simulink model "powersystemsFinalTest"  (R2023a)
settings: Solver=VariableStepAuto  StartTime=0.0  StopTime=50  RelTol=1e-3
model workspace (MAT data in the model file):
  step = 1
values from neighbouring files (symbols this model uses):
  C_TCSC = 1 / (2*pi*60*Xc)    [Final_TCSC.m]
  final_step = [1,1,1,1]    [Final_TCSC.m]
  L_line = X_line / (2*pi*60)    [Final_TCSC.m]
  L_TCSC = Xl_stage / (2*pi*60)    [Final_TCSC.m]
  R_load = 1000    [Final_TCSC.m]
  Vs = str2double(inputs{1}) * 1e3    [Final_TCSC.m]
libraries: spsSeriesRLCBranchLib x10, spsThyristorLib x8, spsRMSLib x7, spsFourierLib x3, spsVoltageMeasurementLib x3, spsPowerLib x2, spsACVoltageSourceLib x1, aerolibconvert2 x1, spsCurrentMeasurementLib x1, sps_lib x1, spspowerguiLib x1
settings Model: Creator=moham  LastModifiedBy=nonyf
settings DebuggingCC: UnconnectedInputMsg=warning  UnconnectedOutputMsg=warning  UnconnectedLineMsg=warning
settings ModelReferenceCC: EnableRefExpFcnMdlSchedulingChecks=on
settings RTWCC: DLArmComputeVersion=19.05

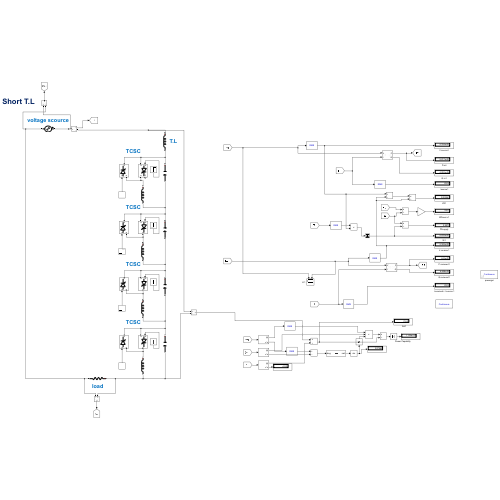
[thumbnail: Simulink's stored preview of the top-level diagram]
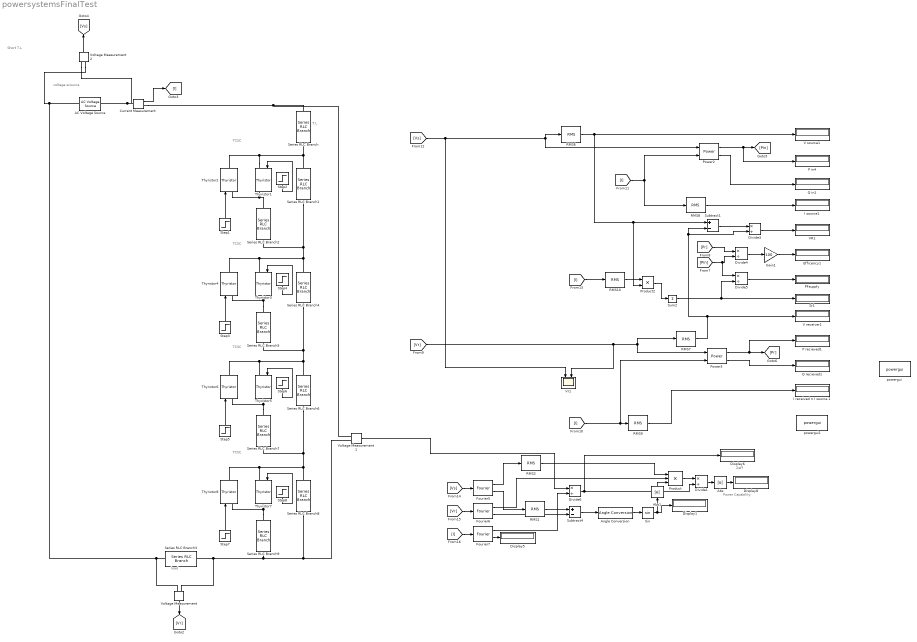
== system powersystemsFinalTest ==
  note: Zeff
  note: load
  note: TCSC
  note: T.L
  note: voltage scource
  note: Short T.L
  note: TCSC
  note: TCSC
  note: TCSC
  note: Power Capability
  AC Voltage Source : spsACVoltageSourceLib/AC Voltage Source  Amplitude=Vs  Phase=0  Frequency=60  SampleTime=0  Measurements=None  BusType=swing  Pref=10e3  Qref=0  Qmin=-inf  Qmax=+inf
  Abs : Abs  SaturateOnIntegerOverflow=off
  Abs1 : Abs  SaturateOnIntegerOverflow=off
  Angle Conversion : aerolibconvert2/Angle Conversion  IU=deg  OU=rad
  Current Measurement : spsCurrentMeasurementLib/Current Measurement  PhasorSimulation=off  OutputType=Complex  PSBequivalent=0
  Display{1,5..6,8} (4 alike) : Display
  Divide{1,3..6} (5 alike) : Product  Inputs=*/
  Efficency1 : Display
  Fourier5 : spsFourierLib/Fourier  Freq=60  n=1  InInit=[0, 0]  Ts=0
  Fourier6 : spsFourierLib/Fourier  Freq=60  n=1  InInit=[0, 0]  Ts=0
  Fourier7 : spsFourierLib/Fourier  Freq=60  n=1  InInit=[0, 0]  Ts=0
  Gain1 : Gain  Gain=100
  I received = I source 1 : Display
  I source1 : Display
  P in4 : Display
  P recieved1 : Display
  PFsupply : Display
  Power2 : spsPowerLib/Power  Freq=60  Vinit=[1, 0]  Iinit=[1, 0]  Ts=0
  Power3 : spsPowerLib/Power  Freq=60  Vinit=[1, 0]  Iinit=[1, 0]  Ts=0
  Product : Product  Inputs=3
  Product2 : Product
  Q in1 : Display
  Q recieved1 : Display
  RMS{1..2,6..10} (7 alike) : spsRMSLib/RMS  TrueRMS=on  Freq=60  RMSInit=120  Ts=0
  Series RLC Branch : spsSeriesRLCBranchLib/Series RLC Branch  LConnTagsString=__new0  RConnTagsString=__new0  BranchType=L  Resistance=50  Inductance=L_line  SetiL0=off  InitialCurrent=0  Capacitance=0  Setx0=off  InitialVoltage=0  Measurements=None
  Series RLC Branch{1,4,6,8} (4 alike) : spsSeriesRLCBranchLib/Series RLC Branch  LConnTagsString=__new0  RConnTagsString=__new0  BranchType=C  Resistance=50  Inductance=0.1327  SetiL0=off  InitialCurrent=0  Capacitance=C_TCSC  Setx0=off  InitialVoltage=0  Measurements=None
  Series RLC Branch{2,5,7,9} (4 alike) : spsSeriesRLCBranchLib/Series RLC Branch  LConnTagsString=__new0  RConnTagsString=__new0  BranchType=L  Resistance=50  Inductance=L_TCSC  SetiL0=off  InitialCurrent=0  Capacitance=0  Setx0=off  InitialVoltage=0  Measurements=None
  Series RLC Branch3 : spsSeriesRLCBranchLib/Series RLC Branch  LConnTagsString=__new0  RConnTagsString=__new0  BranchType=R  Resistance=R_load  Inductance=1.3  SetiL0=off  InitialCurrent=0  Capacitance=0  Setx0=off  InitialVoltage=0  Measurements=None
  Sin : Trigonometry
  Sr1 : Display
  Step1 : Step  Time=5  After=final_step(1)  SampleTime=0
  Step2 : Step  Time=5  After=final_step(1)  SampleTime=0
  Step3 : Step  Time=5  After=final_step(2)  SampleTime=0
  Step4 : Step  Time=5  After=final_step(2)  SampleTime=0  ZeroCross=off
  Step5 : Step  Time=5  After=final_step(3)  SampleTime=0
  Step6 : Step  Time=5  After=final_step(3)  SampleTime=0
  Step7 : Step  Time=5  After=final_step(4)  SampleTime=0
  Step8 : Step  Time=5  After=final_step(4)  SampleTime=0
  Subtract1 : Sum  Inputs=+-
  Subtract4 : Sum  Inputs=+-
  Sum2 : Sum  Inputs=+
  Thyristor1 : spsThyristorLib/Thyristor  Ron=0  Lon=0  Vf=0  IC=0  Rs=0  Cs=0  Measurements=on
  Thyristor{2..8} (7 alike) : spsThyristorLib/Thyristor  Ron=0  Lon=0  Vf=0  IC=0  Rs=0  Cs=0  Measurements=off
  V receiver1 : Display
  V source1 : Display
  VR1 : Display
  Voltage Measurement : spsVoltageMeasurementLib/Voltage Measurement  PhasorSimulation=off  OutputType=Complex  PSBequivalent=0
  Voltage Measurement1 : spsVoltageMeasurementLib/Voltage Measurement  PhasorSimulation=off  OutputType=Complex  PSBequivalent=0
  Voltage Measurement2 : spsVoltageMeasurementLib/Voltage Measurement  PhasorSimulation=off  OutputType=Complex  PSBequivalent=0
  Vr1 : Scope  NumInputPorts=2
  powergui : sps_lib/powergui  Priority=1  SimulationMode=Continuous  SampleTime=50e-6  frequency=60  Iterations=50  frequencyindice=60  Pbase=100e6  ErrMax=1e-4  UnitsV=kV  UnitsW=MW  buscounter=0  FunctionMessages=off  echomessages=off  EnableUseOfTLC=off  CurrentSourceSwitches=off  DisableSnubberDevices=off  DisableRonSwitches=off  DisableVfSwitches=off  DisplayEquations=off  AutomaticDiscreteSolvers=off  SolverType=Tustin/Backward Euler (TBE)  Interpol=off  ExternalGateDelay=off  methode=off  Ts=100  x0status=blocks  SPID=on  SwTol=0  HookPort=off  NonlinearTolerance=1e-4  nMaxIteration=100  ContinueOnMaxIteration=off  RestoreLinks=warning  ResistiveCurrentMeasurement=off  Frange=[0:2:500]  Ylog=off  Xlog=on  ShowGrid=off  save=off  variable=ZData  structure=0  ZoomFFT=off  StartTime=0.0  cycles=1  DisplayStyle=1  fundamental=60  FreqAxis=off  MaxFrequency=1000  frequencyindicesteady=1  RmsSteady=1  display=off
  powergui1 : spspowerguiLib/powergui  Priority=1  SimulationMode=Continuous  SampleTime=50e-6  frequency=60  Iterations=50  frequencyindice=60  Pbase=100e6  ErrMax=1e-4  UnitsV=kV  UnitsW=MW  buscounter=0  FunctionMessages=off  echomessages=off  EnableUseOfTLC=off  CurrentSourceSwitches=off  DisableSnubberDevices=off  DisableRonSwitches=off  DisableVfSwitches=off  DisplayEquations=off  AutomaticDiscreteSolvers=off  SolverType=Tustin/Backward Euler (TBE)  Interpol=off  ExternalGateDelay=off  methode=off  Ts=100  x0status=blocks  SPID=on  SwTol=0  HookPort=off  NonlinearTolerance=1e-4  nMaxIteration=100  ContinueOnMaxIteration=off  RestoreLinks=warning  ResistiveCurrentMeasurement=off  Frange=[0:2:500]  Ylog=off  Xlog=on  ShowGrid=off  save=off  variable=ZData  structure=0  ZoomFFT=off  StartTime=0.0  cycles=1  DisplayStyle=1  fundamental=60  FreqAxis=off  MaxFrequency=1000  frequencyindicesteady=1  RmsSteady=1  display=off
  wires:
  Step1/1 -> Thyristor2/1
  Step2/1 -> Thyristor1/1
  Voltage Measurement/1 -> [Vr]
  Current Measurement/1 -> [I]
  Voltage Measurement2/1 -> [Vs]
  Step3/1 -> Thyristor4/1
  Step4/1 -> Thyristor3/1
  Step6/1 -> Thyristor5/1
  Step5/1 -> Thyristor6/1
  Step8/1 -> Thyristor7/1
  Step7/1 -> Thyristor8/1
  [Vr] -> Fourier6/1
  Fourier7/1 -> Divide6/2
  [I] -> Fourier7/1
  Divide6/1 -> Divide1/2, Display6/1
  [Vs] -> Fourier5/1
  Fourier7/2 -> Display5/1
  Gain1/1 -> Efficency1/1
  Product2/1 -> Sum2/1
  [I] -> Power3/2, RMS9/1
  RMS8/1 -> I source1/1
  Divide3/1 -> VR1/1
  Divide5/1 -> PFsupply/1
  Power3/1 -> P recieved1/1, [Pr]
  RMS10/1 -> Product2/1
  RMS7/1 -> Divide3/2, Subtract1/2, V receiver1/1
  [Pin] -> Divide5/1, Divide4/2
  [Vr] -> RMS7/1, Power3/1, Vr1/2
  RMS9/1 -> I received = I source 1/1
  [Pr] -> Divide4/1
  Power2/1 -> P in4/1, [Pin]
  [I] -> RMS10/1
  Power3/2 -> Q recieved1/1
  Sum2/1 -> Divide5/2, Sr1/1
  Power2/2 -> Q in1/1
  RMS6/1 -> Product2/2, Subtract1/1, V source1/1
  [Vs] -> Power2/1, RMS6/1, Vr1/1
  Subtract1/1 -> Divide3/1
  Divide4/1 -> Gain1/1
  [I] -> RMS8/1, Power2/2
  Fourier5/2 -> RMS1/1
  Fourier6/2 -> Subtract4/2
  Fourier6/1 -> Product/2
  Fourier5/1 -> RMS2/1
  Product/1 -> Divide1/1
  Divide1/1 -> Abs/1
  Abs/1 -> Display8/1
  Voltage Measurement1/1 -> Divide6/1
  Angle Conversion/1 -> Sin/1
  Subtract4/1 -> Angle Conversion/1
  Sin/1 -> Abs1/1, Display1/1
  RMS2/1 -> Product/1
  RMS1/1 -> Subtract4/1
  Abs1/1 -> Product/3
  connections:
  Series RLC Branch4/LConn1 -- Series RLC Branch1/RConn1 -- Series RLC Branch2/RConn1 -- Thyristor4/RConn1 -- Thyristor3/LConn1
  Thyristor1/LConn1 -- Thyristor2/RConn1 -- Series RLC Branch1/LConn1 -- Series RLC Branch/RConn1
  Thyristor1/RConn1 -- Series RLC Branch2/LConn1 -- Thyristor2/LConn1
  Current Measurement/LConn1 -- Voltage Measurement2/LConn1 -- AC Voltage Source/RConn1
  Voltage Measurement/LConn1 -- Voltage Measurement1/LConn2 -- Series RLC Branch8/RConn1 -- Series RLC Branch9/RConn1 -- Series RLC Branch3/LConn1
  Series RLC Branch5/LConn1 -- Thyristor4/LConn1 -- Thyristor3/RConn1
  Series RLC Branch6/LConn1 -- Series RLC Branch4/RConn1 -- Series RLC Branch5/RConn1 -- Thyristor6/RConn1 -- Thyristor5/LConn1
  Series RLC Branch7/LConn1 -- Thyristor6/LConn1 -- Thyristor5/RConn1
  Series RLC Branch9/LConn1 -- Thyristor8/LConn1 -- Thyristor7/RConn1
  Series RLC Branch6/RConn1 -- Series RLC Branch8/LConn1 -- Thyristor8/RConn1 -- Thyristor7/LConn1 -- Series RLC Branch7/RConn1
  Current Measurement/RConn1 -- Voltage Measurement1/LConn1 -- Series RLC Branch/LConn1
  Voltage Measurement2/LConn2 -- Voltage Measurement/LConn2 -- Series RLC Branch3/RConn1 -- AC Voltage Source/LConn1
